simulink model "main"  (R2023b)
settings: Solver=FixedStepDiscrete  StartTime=0.0  StopTime=inf  FixedStep=0.1  RelTol=1e-3
libraries: simulink x23, hdlsllib x16
settings Model: Creator=RDONASC1  LastModifiedBy=RDONASC1
settings OptimizationCC: DefaultParameterBehavior=Inlined  OptimizeBlockIOStorage=off  EnhancedBackFolding=on  PassReuseOutputArgsThreshold=0  OptimizeDataStoreBuffers=off  BusAssignmentInplaceUpdate=off
settings DebuggingCC: ParameterTunabilityLossMsg=error  SFUnexpectedBacktrackingDiag=warning  SFNoUnconditionalDefaultTransitionDiag=warning
settings SFSimCC: MATLABDynamicMemAlloc=off
settings RTWCC: GenerateReport=on  BuildConfiguration=Debug  LaunchReport=on
settings CodeAppCC: ForceParamTrailComments=on  OperatorAnnotations=on  MATLABSourceComments=on  EnableCustomComments=on
settings GRTTargetCC: CombineSignalStateStructs=on  SupportVariableSizeSignals=on  MultiInstanceErrorCode=Warning

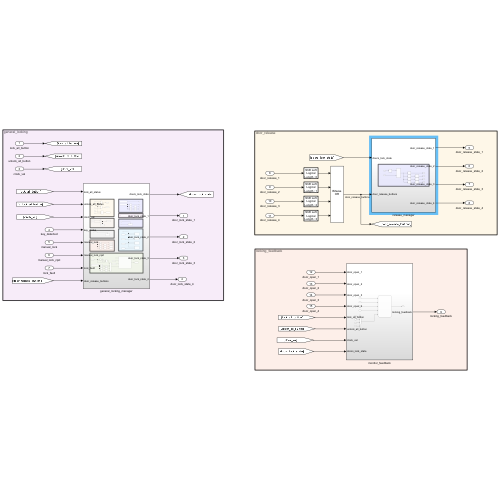
[thumbnail: Simulink's stored preview of the top-level diagram]
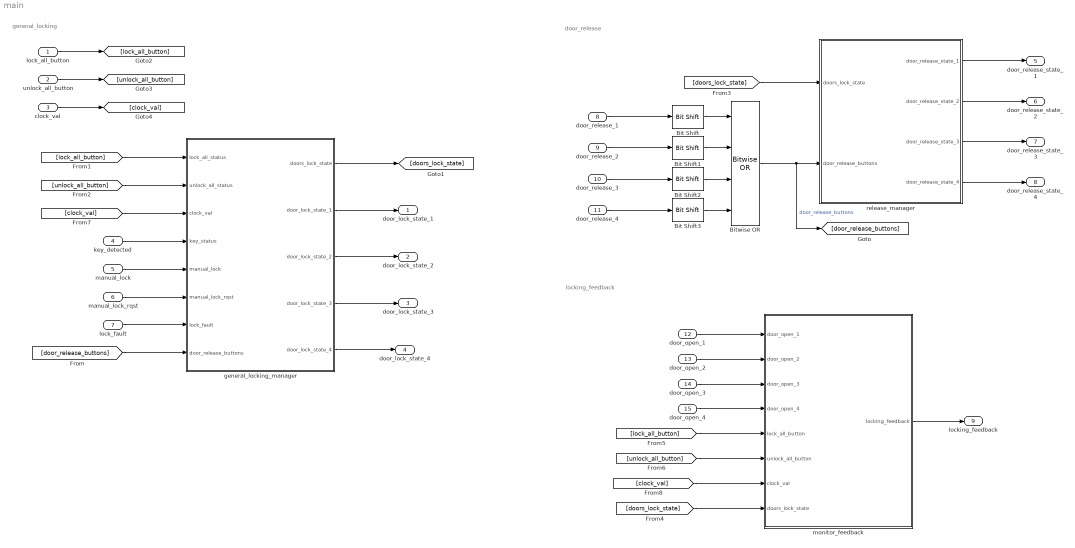
== system main ==
  note: door_release
  note: locking_feedback
  note: general_locking
  lock_all_button : Inport  OutDataTypeStr=uint8
  unlock_all_button : Inport  Port=2  OutDataTypeStr=uint8
  clock_val : Inport  Port=3  OutDataTypeStr=uint64
  key_detected : Inport  Port=4  OutDataTypeStr=uint8
  manual_lock : Inport  Port=5  OutDataTypeStr=uint8
  manual_lock_rqst : Inport  Port=6  OutDataTypeStr=uint8
  lock_fault : Inport  Port=7  OutDataTypeStr=uint8
  door_release_1 : Inport  Port=8  OutDataTypeStr=uint8
  door_release_2 : Inport  Port=9  OutDataTypeStr=uint8
  door_release_3 : Inport  Port=10  OutDataTypeStr=uint8
  door_release_4 : Inport  Port=11  OutDataTypeStr=uint8
  door_open_1 : Inport  Port=12  OutDataTypeStr=uint8
  door_open_2 : Inport  Port=13  OutDataTypeStr=uint8
  door_open_3 : Inport  Port=14  OutDataTypeStr=uint8
  door_open_4 : Inport  Port=15  OutDataTypeStr=uint8
  Bit Shift : hdlsllib/Logic and Bit Operations/Bit Shift  mode=Shift Left Logical  N=0
  Bit Shift1 : hdlsllib/Logic and Bit Operations/Bit Shift  mode=Shift Left Logical  N=1
  Bit Shift2 : hdlsllib/Logic and Bit Operations/Bit Shift  mode=Shift Left Logical  N=2
  Bit Shift3 : hdlsllib/Logic and Bit Operations/Bit Shift  mode=Shift Left Logical  N=3
  Bitwise OR : simulink/Logic and Bit Operations/Bitwise Operator  logicop=OR  UseBitMask=off  NumInputPorts=4  BitMask=bin2dec('11011001')  BitMaskRealWorld=Stored Integer
      settings: LibrarySourceBlock=|
      | simulink/Quick Insert/Logic and Bit
      | Operations/Bitwise OR
  general_locking_manager : Subsystem
  monitor_feedback : Subsystem
  release_manager : Subsystem
  door_lock_state_1 : Outport  OutDataTypeStr=uint8
  door_lock_state_2 : Outport  Port=2  OutDataTypeStr=uint8
  door_lock_state_3 : Outport  Port=3  OutDataTypeStr=uint8
  door_lock_state_4 : Outport  Port=4  OutDataTypeStr=uint8
  door_release_state_1 : Outport  Port=5  OutDataTypeStr=uint8
  door_release_state_2 : Outport  Port=6  OutDataTypeStr=uint8
  door_release_state_3 : Outport  Port=7  OutDataTypeStr=uint8
  door_release_state_4 : Outport  Port=8  OutDataTypeStr=uint8
  locking_feedback : Outport  Port=9  OutDataTypeStr=uint8
  wires:
  door_release_1/1 -> Bit Shift/1
  door_release_2/1 -> Bit Shift1/1
  door_release_3/1 -> Bit Shift2/1
  door_release_4/1 -> Bit Shift3/1
  Bitwise OR/1 -> [door_release_buttons], release_manager/2(door_release_buttons)  "door_release_buttons"
  Bit Shift/1 -> Bitwise OR/1
  Bit Shift1/1 -> Bitwise OR/2
  Bit Shift2/1 -> Bitwise OR/3
  Bit Shift3/1 -> Bitwise OR/4
  release_manager/1(door_release_state_1) -> door_release_state_1/1
  key_detected/1 -> general_locking_manager/4(key_status)
  [door_release_buttons] -> general_locking_manager/8(door_release_buttons)
  lock_fault/1 -> general_locking_manager/7(lock_fault)
  manual_lock/1 -> general_locking_manager/5(manual_lock)
  [doors_lock_state] -> release_manager/1(doors_lock_state)
  door_open_1/1 -> monitor_feedback/1(door_open_1)
  door_open_2/1 -> monitor_feedback/2(door_open_2)
  door_open_3/1 -> monitor_feedback/3(door_open_3)
  door_open_4/1 -> monitor_feedback/4(door_open_4)
  [doors_lock_state] -> monitor_feedback/8(doors_lock_state)
  monitor_feedback/1(locking_feedback) -> locking_feedback/1
  general_locking_manager/1(doors_lock_state) -> [doors_lock_state]
  general_locking_manager/2(door_lock_state_1) -> door_lock_state_1/1
  general_locking_manager/5(door_lock_state_4) -> door_lock_state_4/1
  general_locking_manager/4(door_lock_state_3) -> door_lock_state_3/1
  general_locking_manager/3(door_lock_state_2) -> door_lock_state_2/1
  release_manager/4(door_release_state_4) -> door_release_state_4/1
  release_manager/3(door_release_state_3) -> door_release_state_3/1
  release_manager/2(door_release_state_2) -> door_release_state_2/1
  manual_lock_rqst/1 -> general_locking_manager/6(manual_lock_rqst)
  lock_all_button/1 -> [lock_all_button]
  unlock_all_button/1 -> [unlock_all_button]
  [unlock_all_button] -> general_locking_manager/2(unlock_all_status)
  [lock_all_button] -> general_locking_manager/1(lock_all_status)
  [lock_all_button] -> monitor_feedback/5(lock_all_button)
  [unlock_all_button] -> monitor_feedback/6(unlock_all_button)
  clock_val/1 -> [clock_val]
  [clock_val] -> general_locking_manager/3(clock_val)
  [clock_val] -> monitor_feedback/7(clock_val)

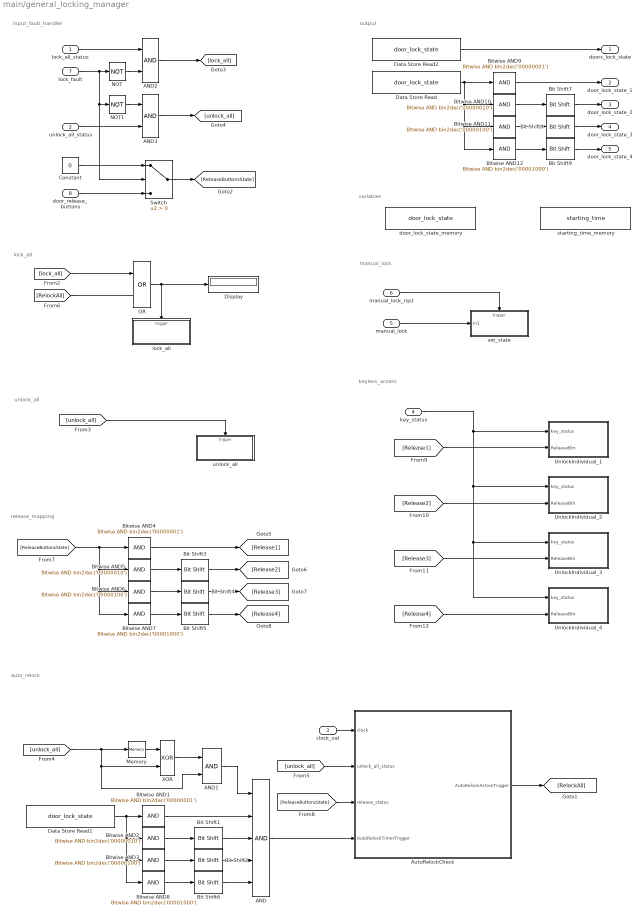
== system main/general_locking_manager ==
  note: input_fault_handler
  note: output
  note: manual_lock
  note: variables
  note: auto_relock
  note: keyless_access
  note: release_mapping
  note: unlock_all
  note: lock_all
  lock_all_status : Inport
  unlock_all_status : Inport  Port=2
  clock_val : Inport  Port=3
  key_status : Inport  Port=4
  manual_lock : Inport  Port=5
  manual_lock_rqst : Inport  Port=6
  lock_fault : Inport  Port=7
  door_release_buttons : Inport  Port=8
  AND : Logic  Inputs=5  IconShape=distinctive  AllPortsSameDT=off  OutDataTypeStr=boolean
  AND1 : Logic  IconShape=distinctive  AllPortsSameDT=off  OutDataTypeStr=boolean
  AND2 : Logic  IconShape=distinctive  AllPortsSameDT=off  OutDataTypeStr=boolean
  AND3 : Logic  IconShape=distinctive  AllPortsSameDT=off  OutDataTypeStr=boolean
  AutoRelockCheck : Stateflow chart  TreatAsAtomicUnit=on
  Bit Shift1 : hdlsllib/Logic and Bit Operations/Bit Shift  mode=Shift Right Logical  N=1
  Bit Shift2 : hdlsllib/Logic and Bit Operations/Bit Shift  mode=Shift Right Logical  N=2
  Bit Shift3 : hdlsllib/Logic and Bit Operations/Bit Shift  mode=Shift Right Logical  N=1
  Bit Shift4 : hdlsllib/Logic and Bit Operations/Bit Shift  mode=Shift Right Logical  N=2
  Bit Shift5 : hdlsllib/Logic and Bit Operations/Bit Shift  mode=Shift Right Logical  N=3
  Bit Shift6 : hdlsllib/Logic and Bit Operations/Bit Shift  mode=Shift Right Logical  N=3
  Bit Shift7 : hdlsllib/Logic and Bit Operations/Bit Shift  mode=Shift Right Logical  N=1
  Bit Shift8 : hdlsllib/Logic and Bit Operations/Bit Shift  mode=Shift Right Logical  N=2
  Bit Shift9 : hdlsllib/Logic and Bit Operations/Bit Shift  mode=Shift Right Logical  N=3
  Bitwise AND1 : simulink/Logic and Bit Operations/Bitwise Operator  logicop=AND  UseBitMask=on  BitMask=bin2dec('00000001')  BitMaskRealWorld=Stored Integer
      settings: LibrarySourceBlock=|
      | simulink/Quick Insert/Logic and Bit
      | Operations/Bitwise AND
  Bitwise AND10 : simulink/Logic and Bit Operations/Bitwise Operator  logicop=AND  UseBitMask=on  BitMask=bin2dec('00000010')  BitMaskRealWorld=Stored Integer
      settings: LibrarySourceBlock=|
      | simulink/Quick Insert/Logic and Bit
      | Operations/Bitwise AND
  Bitwise AND11 : simulink/Logic and Bit Operations/Bitwise Operator  logicop=AND  UseBitMask=on  BitMask=bin2dec('00000100')  BitMaskRealWorld=Stored Integer
      settings: LibrarySourceBlock=|
      | simulink/Quick Insert/Logic and Bit
      | Operations/Bitwise AND
  Bitwise AND12 : simulink/Logic and Bit Operations/Bitwise Operator  logicop=AND  UseBitMask=on  BitMask=bin2dec('00001000')  BitMaskRealWorld=Stored Integer
      settings: LibrarySourceBlock=|
      | simulink/Quick Insert/Logic and Bit
      | Operations/Bitwise AND
  Bitwise AND2 : simulink/Logic and Bit Operations/Bitwise Operator  logicop=AND  UseBitMask=on  BitMask=bin2dec('00000010')  BitMaskRealWorld=Stored Integer
      settings: LibrarySourceBlock=|
      | simulink/Quick Insert/Logic and Bit
      | Operations/Bitwise AND
  Bitwise AND3 : simulink/Logic and Bit Operations/Bitwise Operator  logicop=AND  UseBitMask=on  BitMask=bin2dec('00000100')  BitMaskRealWorld=Stored Integer
      settings: LibrarySourceBlock=|
      | simulink/Quick Insert/Logic and Bit
      | Operations/Bitwise AND
  Bitwise AND4 : simulink/Logic and Bit Operations/Bitwise Operator  logicop=AND  UseBitMask=on  BitMask=bin2dec('00000001')  BitMaskRealWorld=Stored Integer
      settings: LibrarySourceBlock=|
      | simulink/Quick Insert/Logic and Bit
      | Operations/Bitwise AND
  Bitwise AND5 : simulink/Logic and Bit Operations/Bitwise Operator  logicop=AND  UseBitMask=on  BitMask=bin2dec('00000010')  BitMaskRealWorld=Stored Integer
      settings: LibrarySourceBlock=|
      | simulink/Quick Insert/Logic and Bit
      | Operations/Bitwise AND
  Bitwise AND6 : simulink/Logic and Bit Operations/Bitwise Operator  logicop=AND  UseBitMask=on  BitMask=bin2dec('00000100')  BitMaskRealWorld=Stored Integer
      settings: LibrarySourceBlock=|
      | simulink/Quick Insert/Logic and Bit
      | Operations/Bitwise AND
  Bitwise AND7 : simulink/Logic and Bit Operations/Bitwise Operator  logicop=AND  UseBitMask=on  BitMask=bin2dec('00001000')  BitMaskRealWorld=Stored Integer
      settings: LibrarySourceBlock=|
      | simulink/Quick Insert/Logic and Bit
      | Operations/Bitwise AND
  Bitwise AND8 : simulink/Logic and Bit Operations/Bitwise Operator  logicop=AND  UseBitMask=on  BitMask=bin2dec('00001000')  BitMaskRealWorld=Stored Integer
      settings: LibrarySourceBlock=|
      | simulink/Quick Insert/Logic and Bit
      | Operations/Bitwise AND
  Bitwise AND9 : simulink/Logic and Bit Operations/Bitwise Operator  logicop=AND  UseBitMask=on  BitMask=bin2dec('00000001')  BitMaskRealWorld=Stored Integer
      settings: LibrarySourceBlock=|
      | simulink/Quick Insert/Logic and Bit
      | Operations/Bitwise AND
  Constant : Constant  Value=0  OutDataTypeStr=uint8
  Data Store Read : DataStoreRead  DataStoreName=door_lock_state  IndexOptions=Index vector (dialog)  Indices=1  OutputSizes=1
  Data Store Read1 : DataStoreRead  DataStoreName=door_lock_state  IndexOptions=Index vector (dialog)  Indices=1  OutputSizes=1
  Data Store Read2 : DataStoreRead  DataStoreName=door_lock_state  IndexOptions=Index vector (dialog)  Indices=1  OutputSizes=1
  Display : Display
  Memory : Memory
  NOT : Logic  Operator=NOT  IconShape=distinctive  AllPortsSameDT=off  OutDataTypeStr=boolean
  NOT1 : Logic  Operator=NOT  IconShape=distinctive  AllPortsSameDT=off  OutDataTypeStr=boolean
  OR : Logic  Operator=OR  IconShape=distinctive  AllPortsSameDT=off  OutDataTypeStr=boolean
  Switch : Switch  Criteria=u2 > Threshold  SaturateOnIntegerOverflow=off  InputSameDT=off
  UnlockIndividual_1 : Subsystem
  UnlockIndividual_2 : Subsystem
  UnlockIndividual_3 : Subsystem
  UnlockIndividual_4 : Subsystem
  XOR : Logic  Operator=XOR  IconShape=distinctive  AllPortsSameDT=off  OutDataTypeStr=boolean
  door_lock_state_memory : DataStoreMemory  DataStoreName=door_lock_state  WriteAfterWriteMsg=warning  ShowAdditionalParam=off
  lock_all : Subsystem  TreatAsAtomicUnit=on
  set_state : Subsystem  TreatAsAtomicUnit=on
  starting_time_memory : DataStoreMemory  DataStoreName=starting_time  WriteAfterWriteMsg=warning  ShowAdditionalParam=off  OutDataTypeStr=uint64
  unlock_all : Subsystem  TreatAsAtomicUnit=on
  doors_lock_state : Outport
  door_lock_state_1 : Outport  Port=2
  door_lock_state_2 : Outport  Port=3
  door_lock_state_3 : Outport  Port=4
  door_lock_state_4 : Outport  Port=5
  wires:
  lock_all_status/1 -> AND2/1
  manual_lock/1 -> set_state/1(In1)
  [unlock_all] -> AutoRelockCheck/2(unlock_all_status)
  [ReleaseButtonsState] -> AutoRelockCheck/3(release_status)
  Bit Shift4/1 -> [Release3]
  Bitwise AND7/1 -> Bit Shift5/1
  Bit Shift3/1 -> [Release2]
  Bitwise AND6/1 -> Bit Shift4/1
  Bitwise AND4/1 -> [Release1]
  Bitwise AND5/1 -> Bit Shift3/1
  Bit Shift5/1 -> [Release4]
  [ReleaseButtonsState] -> Bitwise AND7/1, Bitwise AND6/1, Bitwise AND5/1, Bitwise AND4/1
  AND/1 -> AutoRelockCheck/4(AutoRelockTimerTrigger)
  AutoRelockCheck/1(AutoRelockActionTrigger) -> [RelockAll]
  OR/1 -> Display/1, lock_all/Trigger
  [RelockAll] -> OR/2
  [unlock_all] -> AND1/2, XOR/2, Memory/1
  Memory/1 -> XOR/1
  XOR/1 -> AND1/1
  AND1/1 -> AND/1
  [Release1] -> UnlockIndividual_1/2(ReleaseBtn)
  key_status/1 -> UnlockIndividual_4/1(key_status), UnlockIndividual_3/1(key_status), UnlockIndividual_2/1(key_status), UnlockIndividual_1/1(key_status)
  [Release3] -> UnlockIndividual_3/2(ReleaseBtn)
  [Release2] -> UnlockIndividual_2/2(ReleaseBtn)
  [Release4] -> UnlockIndividual_4/2(ReleaseBtn)
  clock_val/1 -> AutoRelockCheck/1(clock)
  Bit Shift6/1 -> AND/5
  Bit Shift1/1 -> AND/3
  Bitwise AND3/1 -> Bit Shift2/1
  Bitwise AND1/1 -> AND/2
  Bitwise AND8/1 -> Bit Shift6/1
  Bit Shift2/1 -> AND/4
  Bitwise AND2/1 -> Bit Shift1/1
  Data Store Read1/1 -> Bitwise AND8/1, Bitwise AND3/1, Bitwise AND2/1, Bitwise AND1/1
  [lock_all] -> OR/1
  [unlock_all] -> unlock_all/Trigger
  Bitwise AND12/1 -> Bit Shift9/1
  Bitwise AND11/1 -> Bit Shift8/1
  Data Store Read/1 -> Bitwise AND12/1, Bitwise AND11/1, Bitwise AND10/1, Bitwise AND9/1
  Bitwise AND10/1 -> Bit Shift7/1
  Bitwise AND9/1 -> door_lock_state_1/1
  Bit Shift7/1 -> door_lock_state_2/1
  Bit Shift8/1 -> door_lock_state_3/1
  Bit Shift9/1 -> door_lock_state_4/1
  Data Store Read2/1 -> doors_lock_state/1
  manual_lock_rqst/1 -> set_state/Trigger
  lock_fault/1 -> Switch/2, NOT1/1, NOT/1
  AND2/1 -> [lock_all]
  NOT/1 -> AND2/2
  NOT1/1 -> AND3/1
  AND3/1 -> [unlock_all]
  unlock_all_status/1 -> AND3/2
  door_release_buttons/1 -> Switch/3
  Constant/1 -> Switch/1
  Switch/1 -> [ReleaseButtonsState]

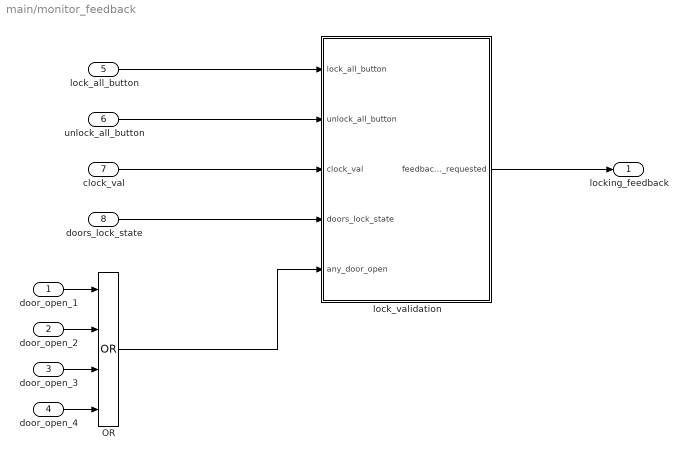
== system main/monitor_feedback ==
  door_open_1 : Inport
  door_open_2 : Inport  Port=2
  door_open_3 : Inport  Port=3
  door_open_4 : Inport  Port=4
  lock_all_button : Inport  Port=5
  unlock_all_button : Inport  Port=6
  clock_val : Inport  Port=7
  doors_lock_state : Inport  Port=8
  OR : Logic  Operator=OR  Inputs=4  IconShape=distinctive  AllPortsSameDT=off  OutDataTypeStr=boolean
  lock_validation : Stateflow chart  TreatAsAtomicUnit=on
      settings: PortSchema="{\"entries\":[{\"content\":{\"sides\":[{\"content\":{\"connectorIds\":[\"In2\",\"In3\",\"In4\",\"In5\",\"In1\"]},\"type\":\"ConnectorPlacement.EquallySpacedRectSide\",\"uuid\":\"52e15686-5ebb-4dff-9781-48c2c4b3ce78\"},{\"content\":{\"connectorIds\":[\"Out1\"],\"side\":\"RIGHT\"},\"type\":\"ConnectorPlacement.EquallySpacedRectSide\",\"uuid\":\"a20341eb-56fb-48bd-b170-7e58cea06054\"},{\"content\":{\"side\":\"TOP\"},\"type\":\"ConnectorPlacement.EquallySpacedRectSide\",\"uuid\":\"38c4557d-4910-4b99-afc5-e39ad6bab763\"}]},\"type\":\"ConnectorPlacement.EquallySpacedConnector\",\"uuid\":\"5e2a6078-f45f-473c-815c-5a40746b0444\"}],\"packageUris\":[\"http://schema.mathworks.com/mf0/Connector/R2020b\"],\"version\":\"1.0\"}"
  locking_feedback : Outport
  wires:
  lock_all_button/1 -> lock_validation/2(lock_all_button)
  clock_val/1 -> lock_validation/4(clock_val)
  doors_lock_state/1 -> lock_validation/5(doors_lock_state)
  lock_validation/1(feedback_requested) -> locking_feedback/1
  unlock_all_button/1 -> lock_validation/3(unlock_all_button)
  OR/1 -> lock_validation/1(any_door_open)
  door_open_1/1 -> OR/1
  door_open_2/1 -> OR/2
  door_open_3/1 -> OR/3
  door_open_4/1 -> OR/4

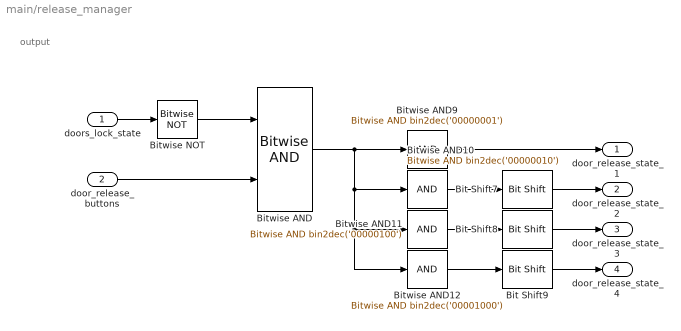
== system main/release_manager ==
  note: output
  doors_lock_state : Inport
  door_release_buttons : Inport  Port=2
  Bit Shift7 : hdlsllib/Logic and Bit Operations/Bit Shift  mode=Shift Right Logical  N=1
  Bit Shift8 : hdlsllib/Logic and Bit Operations/Bit Shift  mode=Shift Right Logical  N=2
  Bit Shift9 : hdlsllib/Logic and Bit Operations/Bit Shift  mode=Shift Right Logical  N=3
  Bitwise AND : simulink/Logic and Bit Operations/Bitwise Operator  logicop=AND  UseBitMask=off  NumInputPorts=2  BitMask=bin2dec('11011001')  BitMaskRealWorld=Stored Integer
      settings: LibrarySourceBlock=|
      | simulink/Quick Insert/Logic and Bit
      | Operations/Bitwise AND
  Bitwise AND10 : simulink/Logic and Bit Operations/Bitwise Operator  logicop=AND  UseBitMask=on  BitMask=bin2dec('00000010')  BitMaskRealWorld=Stored Integer
      settings: LibrarySourceBlock=|
      | simulink/Quick Insert/Logic and Bit
      | Operations/Bitwise AND
  Bitwise AND11 : simulink/Logic and Bit Operations/Bitwise Operator  logicop=AND  UseBitMask=on  BitMask=bin2dec('00000100')  BitMaskRealWorld=Stored Integer
      settings: LibrarySourceBlock=|
      | simulink/Quick Insert/Logic and Bit
      | Operations/Bitwise AND
  Bitwise AND12 : simulink/Logic and Bit Operations/Bitwise Operator  logicop=AND  UseBitMask=on  BitMask=bin2dec('00001000')  BitMaskRealWorld=Stored Integer
      settings: LibrarySourceBlock=|
      | simulink/Quick Insert/Logic and Bit
      | Operations/Bitwise AND
  Bitwise AND9 : simulink/Logic and Bit Operations/Bitwise Operator  logicop=AND  UseBitMask=on  BitMask=bin2dec('00000001')  BitMaskRealWorld=Stored Integer
      settings: LibrarySourceBlock=|
      | simulink/Quick Insert/Logic and Bit
      | Operations/Bitwise AND
  Bitwise NOT : simulink/Logic and Bit Operations/Bitwise Operator  logicop=NOT  UseBitMask=off  BitMask=bin2dec('11011001')  BitMaskRealWorld=Stored Integer
      settings: LibrarySourceBlock=|
      | simulink/Quick Insert/Logic and Bit
      | Operations/Bitwise NOT
  door_release_state_1 : Outport
  door_release_state_2 : Outport  Port=2
  door_release_state_3 : Outport  Port=3
  door_release_state_4 : Outport  Port=4
  wires:
  doors_lock_state/1 -> Bitwise NOT/1
  Bitwise NOT/1 -> Bitwise AND/1
  door_release_buttons/1 -> Bitwise AND/2
  Bitwise AND9/1 -> door_release_state_1/1
  Bitwise AND11/1 -> Bit Shift8/1
  Bitwise AND12/1 -> Bit Shift9/1
  Bitwise AND/1 -> Bitwise AND12/1, Bitwise AND11/1, Bitwise AND10/1, Bitwise AND9/1
  Bitwise AND10/1 -> Bit Shift7/1
  Bit Shift7/1 -> door_release_state_2/1
  Bit Shift8/1 -> door_release_state_3/1
  Bit Shift9/1 -> door_release_state_4/1

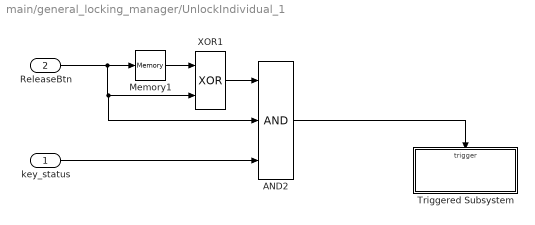
== system main/general_locking_manager/UnlockIndividual_1 ==
  key_status : Inport
  ReleaseBtn : Inport  Port=2
  AND2 : Logic  Inputs=3  IconShape=distinctive  AllPortsSameDT=off  OutDataTypeStr=boolean
  Memory1 : Memory
  Triggered Subsystem : Subsystem  TreatAsAtomicUnit=on
  XOR1 : Logic  Operator=XOR  IconShape=distinctive  AllPortsSameDT=off  OutDataTypeStr=boolean
  wires:
  ReleaseBtn/1 -> AND2/2, XOR1/2, Memory1/1
  key_status/1 -> AND2/3
  XOR1/1 -> AND2/1
  Memory1/1 -> XOR1/1
  AND2/1 -> Triggered Subsystem/Trigger

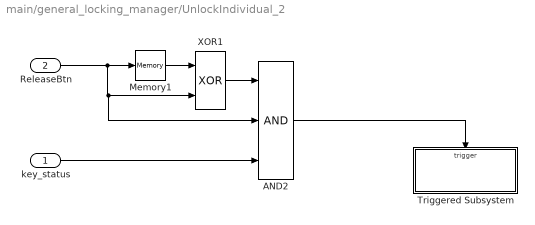
== system main/general_locking_manager/UnlockIndividual_2 ==
  key_status : Inport
  ReleaseBtn : Inport  Port=2
  AND2 : Logic  Inputs=3  IconShape=distinctive  AllPortsSameDT=off  OutDataTypeStr=boolean
  Memory1 : Memory
  Triggered Subsystem : Subsystem  TreatAsAtomicUnit=on
  XOR1 : Logic  Operator=XOR  IconShape=distinctive  AllPortsSameDT=off  OutDataTypeStr=boolean
  wires:
  ReleaseBtn/1 -> AND2/2, XOR1/2, Memory1/1
  key_status/1 -> AND2/3
  XOR1/1 -> AND2/1
  Memory1/1 -> XOR1/1
  AND2/1 -> Triggered Subsystem/Trigger

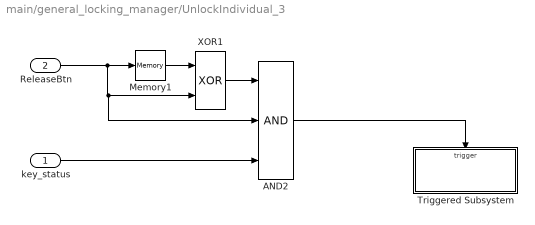
== system main/general_locking_manager/UnlockIndividual_3 ==
  key_status : Inport
  ReleaseBtn : Inport  Port=2
  AND2 : Logic  Inputs=3  IconShape=distinctive  AllPortsSameDT=off  OutDataTypeStr=boolean
  Memory1 : Memory
  Triggered Subsystem : Subsystem  TreatAsAtomicUnit=on
  XOR1 : Logic  Operator=XOR  IconShape=distinctive  AllPortsSameDT=off  OutDataTypeStr=boolean
  wires:
  ReleaseBtn/1 -> AND2/2, XOR1/2, Memory1/1
  key_status/1 -> AND2/3
  XOR1/1 -> AND2/1
  Memory1/1 -> XOR1/1
  AND2/1 -> Triggered Subsystem/Trigger

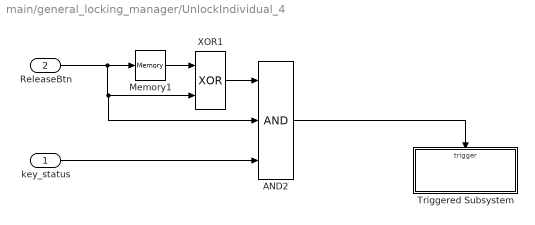
== system main/general_locking_manager/UnlockIndividual_4 ==
  key_status : Inport
  ReleaseBtn : Inport  Port=2
  AND2 : Logic  Inputs=3  IconShape=distinctive  AllPortsSameDT=off  OutDataTypeStr=boolean
  Memory1 : Memory
  Triggered Subsystem : Subsystem  TreatAsAtomicUnit=on
  XOR1 : Logic  Operator=XOR  IconShape=distinctive  AllPortsSameDT=off  OutDataTypeStr=boolean
  wires:
  ReleaseBtn/1 -> AND2/2, XOR1/2, Memory1/1
  key_status/1 -> AND2/3
  XOR1/1 -> AND2/1
  Memory1/1 -> XOR1/1
  AND2/1 -> Triggered Subsystem/Trigger

== system main/general_locking_manager/lock_all ==
  Trigger : TriggerPort  VariantControl=(inherit)
  Constant : Constant  Value=0b00001111  OutDataTypeStr=uint8
  Data Store Write : DataStoreWrite  DataStoreName=door_lock_state  IndexOptions=Index vector (dialog)  Indices=1  OutputSizes=1
  wires:
  Constant/1 -> Data Store Write/1

== system main/general_locking_manager/set_state ==
  In1 : Inport
  Trigger : TriggerPort  VariantControl=(inherit)
  Data Store Write : DataStoreWrite  DataStoreName=door_lock_state  IndexOptions=Index vector (dialog)  Indices=1  OutputSizes=1
  wires:
  In1/1 -> Data Store Write/1

== system main/general_locking_manager/unlock_all ==
  Trigger : TriggerPort  VariantControl=(inherit)
  Constant : Constant  Value=0b00000000  OutDataTypeStr=uint8
  Data Store Write : DataStoreWrite  DataStoreName=door_lock_state  IndexOptions=Index vector (dialog)  Indices=1  OutputSizes=1
  wires:
  Constant/1 -> Data Store Write/1

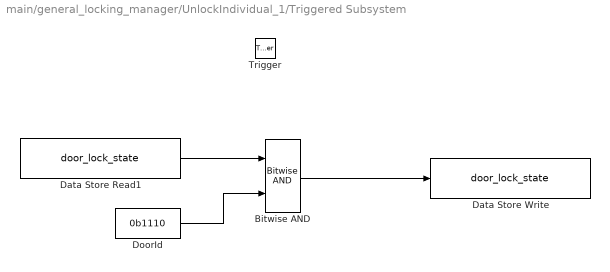
== system main/general_locking_manager/UnlockIndividual_1/Triggered Subsystem ==
  Trigger : TriggerPort  VariantControl=(inherit)
  Bitwise AND : simulink/Logic and Bit Operations/Bitwise Operator  logicop=AND  UseBitMask=off  NumInputPorts=2  BitMask=bin2dec('11011001')  BitMaskRealWorld=Stored Integer
      settings: LibrarySourceBlock=|
      | simulink/Quick Insert/Logic and Bit
      | Operations/Bitwise AND
  Data Store Read1 : DataStoreRead  DataStoreName=door_lock_state  IndexOptions=Index vector (dialog)  Indices=1  OutputSizes=1
  Data Store Write : DataStoreWrite  DataStoreName=door_lock_state  IndexOptions=Index vector (dialog)  Indices=1  OutputSizes=1
  DoorId : Constant  Value=0b1110  OutDataTypeStr=uint8
  wires:
  Data Store Read1/1 -> Bitwise AND/1
  Bitwise AND/1 -> Data Store Write/1
  DoorId/1 -> Bitwise AND/2

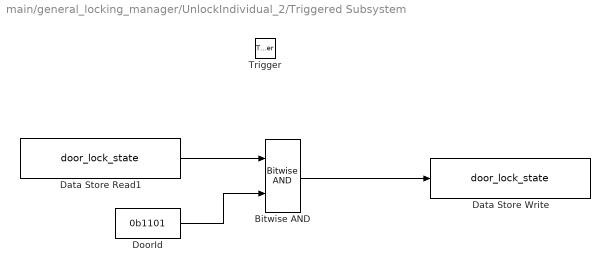
== system main/general_locking_manager/UnlockIndividual_2/Triggered Subsystem ==
  Trigger : TriggerPort  VariantControl=(inherit)
  Bitwise AND : simulink/Logic and Bit Operations/Bitwise Operator  logicop=AND  UseBitMask=off  NumInputPorts=2  BitMask=bin2dec('11011001')  BitMaskRealWorld=Stored Integer
      settings: LibrarySourceBlock=|
      | simulink/Quick Insert/Logic and Bit
      | Operations/Bitwise AND
  Data Store Read1 : DataStoreRead  DataStoreName=door_lock_state  IndexOptions=Index vector (dialog)  Indices=1  OutputSizes=1
  Data Store Write : DataStoreWrite  DataStoreName=door_lock_state  IndexOptions=Index vector (dialog)  Indices=1  OutputSizes=1
  DoorId : Constant  Value=0b1101  OutDataTypeStr=uint8
  wires:
  Data Store Read1/1 -> Bitwise AND/1
  Bitwise AND/1 -> Data Store Write/1
  DoorId/1 -> Bitwise AND/2

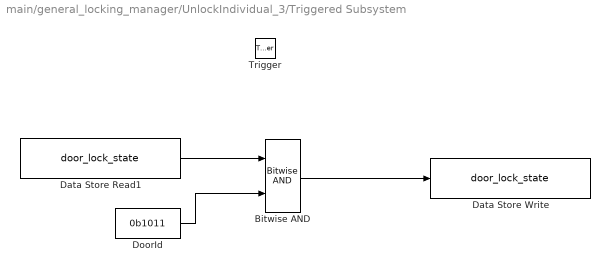
== system main/general_locking_manager/UnlockIndividual_3/Triggered Subsystem ==
  Trigger : TriggerPort  VariantControl=(inherit)
  Bitwise AND : simulink/Logic and Bit Operations/Bitwise Operator  logicop=AND  UseBitMask=off  NumInputPorts=2  BitMask=bin2dec('11011001')  BitMaskRealWorld=Stored Integer
      settings: LibrarySourceBlock=|
      | simulink/Quick Insert/Logic and Bit
      | Operations/Bitwise AND
  Data Store Read1 : DataStoreRead  DataStoreName=door_lock_state  IndexOptions=Index vector (dialog)  Indices=1  OutputSizes=1
  Data Store Write : DataStoreWrite  DataStoreName=door_lock_state  IndexOptions=Index vector (dialog)  Indices=1  OutputSizes=1
  DoorId : Constant  Value=0b1011  OutDataTypeStr=uint8
  wires:
  Data Store Read1/1 -> Bitwise AND/1
  Bitwise AND/1 -> Data Store Write/1
  DoorId/1 -> Bitwise AND/2

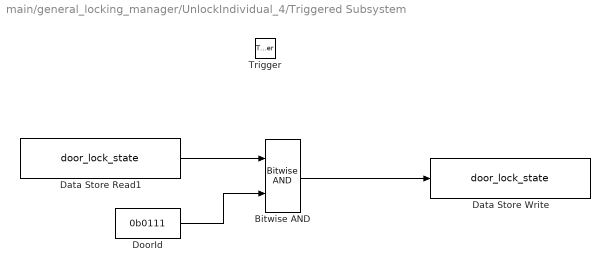
== system main/general_locking_manager/UnlockIndividual_4/Triggered Subsystem ==
  Trigger : TriggerPort  VariantControl=(inherit)
  Bitwise AND : simulink/Logic and Bit Operations/Bitwise Operator  logicop=AND  UseBitMask=off  NumInputPorts=2  BitMask=bin2dec('11011001')  BitMaskRealWorld=Stored Integer
      settings: LibrarySourceBlock=|
      | simulink/Quick Insert/Logic and Bit
      | Operations/Bitwise AND
  Data Store Read1 : DataStoreRead  DataStoreName=door_lock_state  IndexOptions=Index vector (dialog)  Indices=1  OutputSizes=1
  Data Store Write : DataStoreWrite  DataStoreName=door_lock_state  IndexOptions=Index vector (dialog)  Indices=1  OutputSizes=1
  DoorId : Constant  Value=0b0111  OutDataTypeStr=uint8
  wires:
  Data Store Read1/1 -> Bitwise AND/1
  Bitwise AND/1 -> Data Store Write/1
  DoorId/1 -> Bitwise AND/2

== stateflow chart main/general_locking_manager/AutoRelockCheck ==
  state IDLE
    AutoRelockActionTrigger = 0
  state TIMING
    AutoRelockActionTrigger = 0
    state UNLOCK_PRESSED
    state UNLOCK_RELEASED
    (default) -> UNLOCK_PRESSED
    UNLOCK_PRESSED -> UNLOCK_RELEASED : [~unlock_all_status]
  state RELOCK
    AutoRelockActionTrigger = 1
  (default) -> IDLE
  IDLE -> TIMING : [AutoRelockTimerTrigger]{starting_time=clock}
  TIMING -> RELOCK [order 2] : [clock-starting_time > 15000]
  TIMING -> IDLE [order 1] : [release_status > 0]
  RELOCK -> IDLE : [true]
  UNLOCK_RELEASED -> IDLE : [unlock_all_status]
  data: clock input; unlock_all_status input; release_status input; AutoRelockTimerTrigger input; AutoRelockActionTrigger output; starting_time data_store_memory

== stateflow chart main/monitor_feedback/lock_validation ==
  state IDLE
  state lock_requested
    action_time = clock_val
  state lock_validated
    feedback_requested = update_feedback_state(feedback_requested, 1)
  state fault_confirmed
    feedback_requested = update_feedback_state(feedback_requested, 3)
  state unlock_requested
    action_time = clock_val
  state unlock_validated
    feedback_requested = update_feedback_state(feedback_requested, 2)
  lock_validated -> IDLE
  (default) -> IDLE
  fault_confirmed -> IDLE
  IDLE -> lock_requested [order 1] : [lock_all_button > 0 && any_door_open == 0]
  lock_requested -> lock_validated [order 1] : [doors_lock_state == 15]
  IDLE -> fault_confirmed [order 2] : [lock_all_button > 0 && any_door_open > 0]
  unlock_validated -> IDLE
  unlock_requested -> fault_confirmed [order 2] : [clock_val-action_time >= 500]
  lock_requested -> fault_confirmed [order 2] : [clock_val-action_time >= 500]
  IDLE -> unlock_requested [order 3] : [unlock_all_button > 0]
  unlock_requested -> unlock_validated [order 1] : [doors_lock_state == 0]
  data: any_door_open input; lock_all_button input; unlock_all_button input; clock_val input; doors_lock_state input; action_time local; feedback_requested output uint8 =0
